simulink model "Compare_IcestorageWP2Measurement"  (R2018b)
settings: Solver=ode45  StartTime=0  StopTime=(31+29+31+30+31+30+31+14)*24*3600  RelTol=1e-3  EnableMultiTasking=on
undefined symbols (not defined in the file or in its folder): path_carnot
libraries: carnot x39, simulink x4
(part 2 of 2)

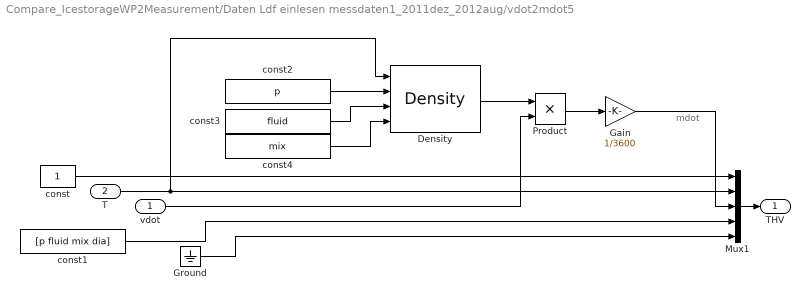
== system Compare_IcestorageWP2Measurement/Daten Ldf einlesen messdaten1_2011dez_2012aug/vdot2mdot5 ==
  note: mdot
  vdot : Inport
  T : Inport  Port=2
  Density : carnot/Basic/Material_Properties/Density  VariantControl=CarlibClassic  INPUTARGUMENTS=state variables (classic)  DEBUGLEVEL=DEBUGLEVEL  MAXTOTALWARNINGS=inf  MAXCONSECUTIVEWARNINGS=inf  WRITETOFILE=0  FILENAME='errors.txt'
      settings: SourceProductName=Carnot
  Gain : Gain  Gain=1/3600
  Ground : Ground
  Mux1 : Mux  Inputs=[1 1 1 4 13]
  Product : Product  RndMeth=Zero
  const : Constant
  const1 : Constant  Value=[p fluid mix dia]
  const2 : Constant  Value=p
  const3 : Constant  Value=fluid
  const4 : Constant  Value=mix
  THV : Outport  InitialOutput=0
  wires:
  Gain/1 -> Mux1/3
  const1/1 -> Mux1/4
  T/1 -> Density/1, Mux1/2
  Ground/1 -> Mux1/5
  const/1 -> Mux1/1
  Mux1/1 -> THV/1
  const2/1 -> Density/2
  const3/1 -> Density/3
  const4/1 -> Density/4
  Density/1 -> Product/1
  vdot/1 -> Product/2
  Product/1 -> Gain/1

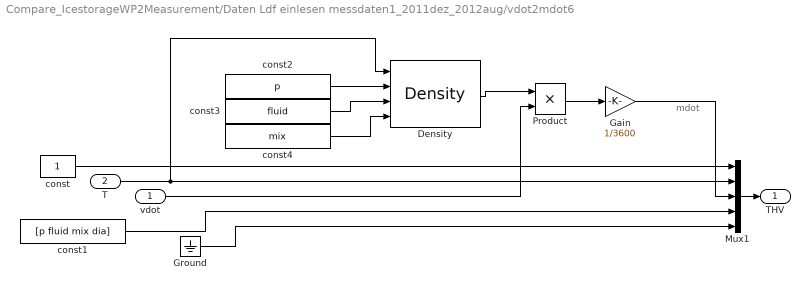
== system Compare_IcestorageWP2Measurement/Daten Ldf einlesen messdaten1_2011dez_2012aug/vdot2mdot6 ==
  note: mdot
  vdot : Inport
  T : Inport  Port=2
  Density : carnot/Basic/Material_Properties/Density  VariantControl=CarlibClassic  INPUTARGUMENTS=state variables (classic)  DEBUGLEVEL=DEBUGLEVEL  MAXTOTALWARNINGS=inf  MAXCONSECUTIVEWARNINGS=inf  WRITETOFILE=0  FILENAME='errors.txt'
      settings: SourceProductName=Carnot
  Gain : Gain  Gain=1/3600
  Ground : Ground
  Mux1 : Mux  Inputs=[1 1 1 4 13]
  Product : Product  RndMeth=Zero
  const : Constant
  const1 : Constant  Value=[p fluid mix dia]
  const2 : Constant  Value=p
  const3 : Constant  Value=fluid
  const4 : Constant  Value=mix
  THV : Outport  InitialOutput=0
  wires:
  Gain/1 -> Mux1/3
  const1/1 -> Mux1/4
  T/1 -> Density/1, Mux1/2
  Ground/1 -> Mux1/5
  const/1 -> Mux1/1
  Mux1/1 -> THV/1
  const2/1 -> Density/2
  const3/1 -> Density/3
  const4/1 -> Density/4
  Density/1 -> Product/1
  vdot/1 -> Product/2
  Product/1 -> Gain/1

== system Compare_IcestorageWP2Measurement/Daten Ldf einlesen messdaten1_2011dez_2012aug/vdot2mdot7 ==
  note: mdot
  vdot : Inport
  T : Inport  Port=2
  Density : carnot/Basic/Material_Properties/Density  VariantControl=CarlibClassic  INPUTARGUMENTS=state variables (classic)  DEBUGLEVEL=DEBUGLEVEL  MAXTOTALWARNINGS=inf  MAXCONSECUTIVEWARNINGS=inf  WRITETOFILE=0  FILENAME='errors.txt'
      settings: SourceProductName=Carnot
  Gain : Gain  Gain=1/3600
  Ground : Ground
  Mux1 : Mux  Inputs=[1 1 1 4 13]
  Product : Product  RndMeth=Zero
  const : Constant
  const1 : Constant  Value=[p fluid mix dia]
  const2 : Constant  Value=p
  const3 : Constant  Value=fluid
  const4 : Constant  Value=mix
  THV : Outport  InitialOutput=0
  wires:
  Product/1 -> Gain/1
  vdot/1 -> Product/2
  Density/1 -> Product/1
  const4/1 -> Density/4
  const3/1 -> Density/3
  const2/1 -> Density/2
  Mux1/1 -> THV/1
  const/1 -> Mux1/1
  Ground/1 -> Mux1/5
  T/1 -> Density/1, Mux1/2
  const1/1 -> Mux1/4
  Gain/1 -> Mux1/3

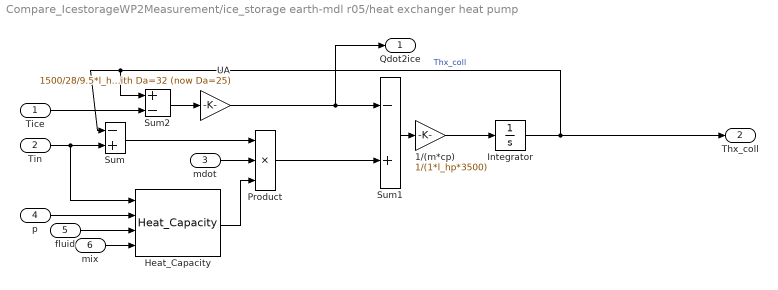
== system Compare_IcestorageWP2Measurement/ice_storage earth-mdl r05/heat exchanger heat pump ==
  Tice : Inport
  Tin : Inport  Port=2
  mdot : Inport  Port=3
  p : Inport  Port=4
  fluid : Inport  Port=5
  mix : Inport  Port=6
  1/(m*cp) : Gain  Gain=1/(1*l_hp*3500)  SaturateOnIntegerOverflow=on  OutDataTypeStr=Inherit: Same as input  ParamDataTypeStr=Inherit: Same as input
  Heat_Capacity : carnot/Basic/Material_Properties/Heat_Capacity  VariantControl=CarlibClassic  INPUTARGUMENTS=state variables (classic)  DEBUGLEVEL=DEBUGLEVEL  MAXTOTALWARNINGS=inf  MAXCONSECUTIVEWARNINGS=inf  WRITETOFILE=0  FILENAME='errors.txt'
      settings: SourceProductName=Carnot
  Integrator : Integrator
  Product : Product  Inputs=3  SaturateOnIntegerOverflow=on  InputSameDT=on  OutDataTypeStr=Inherit: Same as first input
  Sum : Sum  Inputs=-+  SaturateOnIntegerOverflow=on  InputSameDT=on  OutDataTypeStr=Inherit: Same as first input
  Sum1 : Sum  Inputs=-+  SaturateOnIntegerOverflow=on  InputSameDT=on  OutDataTypeStr=Inherit: Same as first input
  Sum2 : Sum  Inputs=+-  SaturateOnIntegerOverflow=on  InputSameDT=on  OutDataTypeStr=Inherit: Same as first input
  UA : Gain  Gain="1500/28/9.5*l_hp*25/32            % 1.5 kW at 9 K on a 28 m tube with Da=32 (now Da=25)"  SaturateOnIntegerOverflow=on  OutDataTypeStr=Inherit: Same as input  ParamDataTypeStr=Inherit: Same as input
  Qdot2ice : Outport
  Thx_coll : Outport  Port=2
  wires:
  Tin/1 -> Heat_Capacity/1, Sum/2
  Integrator/1 -> Sum/1, Sum2/1, Thx_coll/1  "Thx_coll"
  Sum1/1 -> 1/(m*cp)/1
  Product/1 -> Sum1/2
  Heat_Capacity/1 -> Product/3
  Sum/1 -> Product/1
  Sum2/1 -> UA/1
  mdot/1 -> Product/2
  p/1 -> Heat_Capacity/2
  fluid/1 -> Heat_Capacity/3
  mix/1 -> Heat_Capacity/4
  Tice/1 -> Sum2/2
  1/(m*cp)/1 -> Integrator/1
  UA/1 -> Sum1/1, Qdot2ice/1

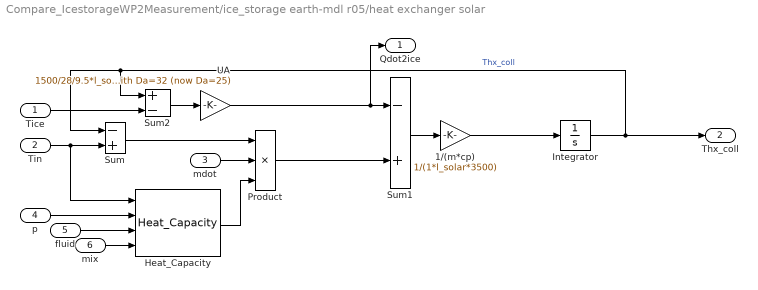
== system Compare_IcestorageWP2Measurement/ice_storage earth-mdl r05/heat exchanger solar ==
  Tice : Inport
  Tin : Inport  Port=2
  mdot : Inport  Port=3
  p : Inport  Port=4
  fluid : Inport  Port=5
  mix : Inport  Port=6
  1/(m*cp) : Gain  Gain=1/(1*l_solar*3500)  SaturateOnIntegerOverflow=on  OutDataTypeStr=Inherit: Same as input  ParamDataTypeStr=Inherit: Same as input
  Heat_Capacity : carnot/Basic/Material_Properties/Heat_Capacity  VariantControl=CarlibClassic  INPUTARGUMENTS=state variables (classic)  DEBUGLEVEL=DEBUGLEVEL  MAXTOTALWARNINGS=inf  MAXCONSECUTIVEWARNINGS=inf  WRITETOFILE=0  FILENAME='errors.txt'
      settings: SourceProductName=Carnot
  Integrator : Integrator
  Product : Product  Inputs=3  SaturateOnIntegerOverflow=on  InputSameDT=on  OutDataTypeStr=Inherit: Same as first input
  Sum : Sum  Inputs=-+  SaturateOnIntegerOverflow=on  InputSameDT=on  OutDataTypeStr=Inherit: Same as first input
  Sum1 : Sum  Inputs=-+  SaturateOnIntegerOverflow=on  InputSameDT=on  OutDataTypeStr=Inherit: Same as first input
  Sum2 : Sum  Inputs=+-  SaturateOnIntegerOverflow=on  InputSameDT=on  OutDataTypeStr=Inherit: Same as first input
  UA : Gain  Gain="1500/28/9.5*l_solar*25/32            % 1.5 kW at 9 K on a 28 m tube with Da=32 (now Da=25)"  SaturateOnIntegerOverflow=on  OutDataTypeStr=Inherit: Same as input  ParamDataTypeStr=Inherit: Same as input
  Qdot2ice : Outport
  Thx_coll : Outport  Port=2
  wires:
  Tice/1 -> Sum2/2
  mix/1 -> Heat_Capacity/4
  fluid/1 -> Heat_Capacity/3
  p/1 -> Heat_Capacity/2
  mdot/1 -> Product/2
  Sum2/1 -> UA/1
  Sum/1 -> Product/1
  Heat_Capacity/1 -> Product/3
  Product/1 -> Sum1/2
  Sum1/1 -> 1/(m*cp)/1
  Integrator/1 -> Thx_coll/1, Sum2/1, Sum/1  "Thx_coll"
  Tin/1 -> Heat_Capacity/1, Sum/2
  1/(m*cp)/1 -> Integrator/1
  UA/1 -> Qdot2ice/1, Sum1/1

== system Compare_IcestorageWP2Measurement/ice_storage earth-mdl r05/undisturbed ground temperature1 ==
  Fcn : Fcn  Expr=u(1) - u(2)*exp(-u(3)/u(4))*cos(2*pi*(u(5)-u(6)*3600)/(365*24*3600) - u(3)/u(4)) + 0.03*u(3)
  Mux : Mux  Inputs=6
  Tmeanoutside : Constant  Value=Tmeanoutside
  delta_grd : Constant  Value=delta_grd
  deltathetae : Constant  Value=deltathetae
  depth of center of wall : Constant  Value=ztilde
  time : Clock
  tshift : Constant  Value=tshift
  Tearth : Outport
  wires:
  Fcn/1 -> Tearth/1
  Mux/1 -> Fcn/1
  tshift/1 -> Mux/6
  time/1 -> Mux/5
  delta_grd/1 -> Mux/4
  depth of center of wall/1 -> Mux/3
  deltathetae/1 -> Mux/2
  Tmeanoutside/1 -> Mux/1
